simulink model "queuetest_third"  (R2018a)
settings: Solver=FixedStepDiscrete  StartTime=0.0  StopTime=10  RelTol=1e-3  EnableMultiTasking=on
model workspace (MAT data in the model file):
  deltat = 0.001
libraries: dspbuff3 x1
settings Model: Creator=The MathWorks, Inc.  LastModifiedBy=Michael Girbino
settings SolverCC: InsertRTBMode=Auto
settings DataIOCC: LimitDataPoints=on  SaveFormat=Array
settings OptimizationCC: ExpressionDepthLimit=2147483647  InitFltsAndDblsToZero=on  LifeSpan=inf
settings DebuggingCC: SaveWithParameterizedLinksMsg=none  UnderspecifiedInitializationDetection=Classic  MergeDetectMultiDrivingBlocksExec=none  SignalResolutionControl=TryResolveAllWithWarning  InheritedTsInSrcMsg=none  MultiTaskDSMMsg=warning  MultiTaskCondExecSysMsg=none  FcnCallInpInsideContextMsg=warning  StateNameClashWarn=warning  SFUnexpectedBacktrackingDiag=warning  SFNoUnconditionalDefaultTransitionDiag=warning  SFExecutionAtInitializationDiag=none
settings HardwareCC: ProdBitPerPointer=32  ProdBitPerSizeT=32  ProdBitPerPtrDiffT=32  ProdLargestAtomicFloat=None  ProdIntDivRoundTo=Undefined  ProdEndianess=Unspecified  ProdWordSize=32  ProdHWDeviceType=32-bit Generic
settings ModelReferenceCC: PropagateSignalLabelsOutOfModel=off
settings SFSimCC: SFSimEcho=off  SimParseCustomCode=off
settings CodeAppCC: StateflowObjectComments=on
settings GRTTargetCC: TargetFcnLib=ansi_tfl_tmw.mat  TargetLangStandard=C89/C90 (ANSI)  GeneratePreprocessorConditionals=Disable all  CombineOutputUpdateFcns=off  GRTInterface=on
settings ConfigComp: CovMetricSettings=dw  CovHtmlReporting=on  CovSaveCumulativeToWorkspaceVar=on  CovSaveSingleToWorkspaceVar=on  CovExternalEMLEnable=off  CovSFcnEnable=off

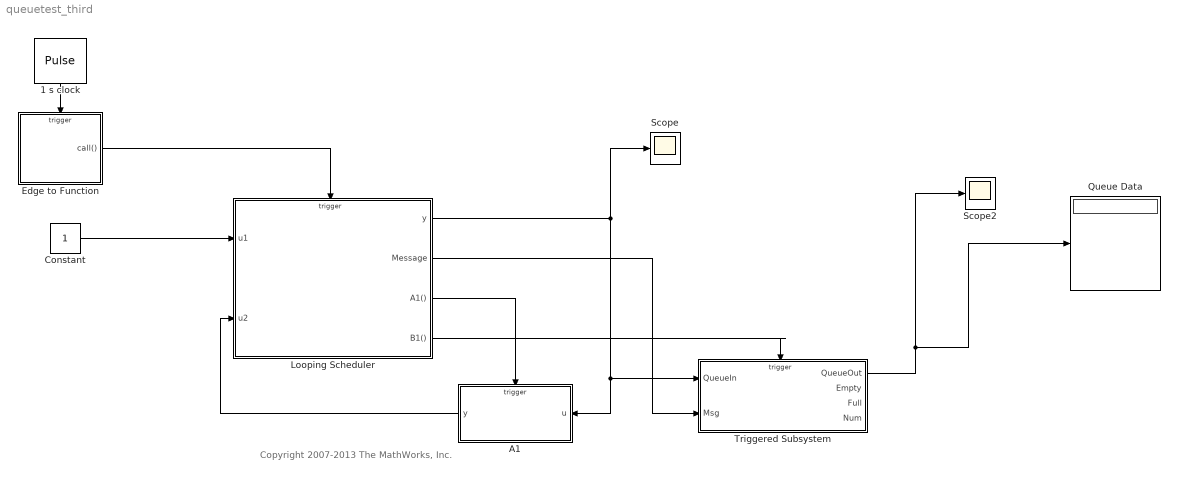
== system queuetest_third ==
  note: Copyright 2007-2013 The MathWorks, Inc.
  1 s clock : DiscretePulseGenerator  PulseType=Time based  Period=1  PulseWidth=10
  A1 : Subsystem  TreatAsAtomicUnit=on
  Constant : Constant
  "Edge to Function " : Stateflow chart  TreatAsAtomicUnit=on
  Looping Scheduler : Stateflow chart  TreatAsAtomicUnit=on
  Queue Data : Display
  Scope : Scope
  Scope2 : Scope
  Triggered Subsystem : Subsystem  TreatAsAtomicUnit=on
  wires:
  Looping Scheduler/1(y) -> Triggered Subsystem/1(QueueIn), A1/1(u), Scope/1
  Looping Scheduler/3(A1()) -> A1/Trigger
  A1/1(y) -> Looping Scheduler/2(u2)
  Constant/1 -> Looping Scheduler/1(u1)
  1 s clock/1 -> "Edge to Function "/Trigger
  "Edge to Function "/1(call()) -> Looping Scheduler/Trigger
  Triggered Subsystem/1(QueueOut) -> Queue Data/1, Scope2/1
  Looping Scheduler/4(B1()) -> Triggered Subsystem/Trigger
  Looping Scheduler/2(Message) -> Triggered Subsystem/2(Msg)

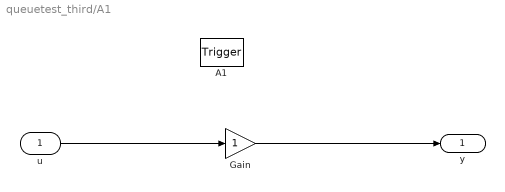
== system queuetest_third/A1 ==
  u : Inport
  A1 : TriggerPort  TriggerType=function-call  VariantControl=Variant
  Gain : Gain
  y : Outport
  wires:
  u/1 -> Gain/1
  Gain/1 -> y/1

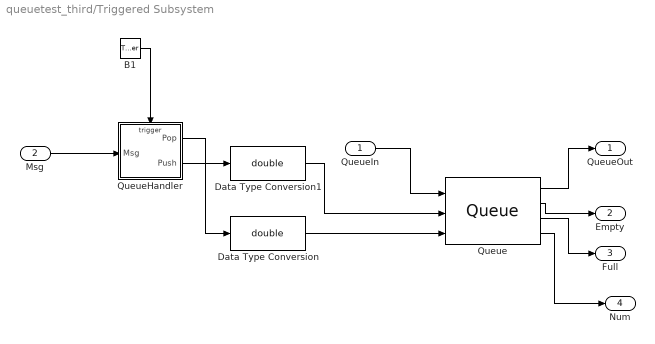
== system queuetest_third/Triggered Subsystem ==
  QueueIn : Inport  OutDataTypeStr=double
  Msg : Inport  Port=2  OutDataTypeStr=double
  B1 : TriggerPort  TriggerType=function-call  VariantControl=Variant  ShowOutputPort=on  OutputDataType=int8  PortDimensions=1
  Data Type Conversion : DataTypeConversion  OutDataTypeStr=double
  Data Type Conversion1 : DataTypeConversion  OutDataTypeStr=double
  Queue : dspbuff3/Queue  depth=8  trigger=Either edge  overflow=Dynamic reallocation  pes=Warning  eso=on  fso=on  nso=on  clr=off  clrOutport=off  adf=on
      settings: SourceProductName=DSP System Toolbox  SourceProductBaseCode=DS
  QueueHandler : Stateflow chart  TreatAsAtomicUnit=on
  QueueOut : Outport  OutDataTypeStr=double
  Empty : Outport  Port=2  OutDataTypeStr=boolean
  Full : Outport  Port=3  OutDataTypeStr=boolean
  Num : Outport  Port=4  OutDataTypeStr=double
  wires:
  QueueIn/1 -> Queue/1
  Queue/1 -> QueueOut/1
  Queue/2 -> Empty/1
  Queue/3 -> Full/1
  Queue/4 -> Num/1
  QueueHandler/1(Pop) -> Data Type Conversion/1
  Data Type Conversion/1 -> Queue/3
  Msg/1 -> QueueHandler/1(Msg)
  B1/1 -> QueueHandler/Trigger
  QueueHandler/2(Push) -> Data Type Conversion1/1
  Data Type Conversion1/1 -> Queue/2

== stateflow chart queuetest_third/Looping Scheduler ==
  (default) -> (junction 5) : {i=1;}
  (junction 6) -> (junction 5) [order 1] : [i<=10]
      | {
      |  y = u1+u2;
      | Message = 1;
      | send(A1);
      | send(B1);
      | i++;
      | }
  (junction 5) -> (junction 6)
  (junction 6) -> (junction 7) [order 2] : // done
  data: y output double; u1 input; u2 input; i local uint32; Message output double
  events: A1 output FUNCTION_CALL_EVENT; call input FUNCTION_CALL_EVENT; B1 output FUNCTION_CALL_EVENT

== stateflow chart queuetest_third/Edge to Function  ==
  (default) -> (junction 2) : {call;}
  events: edge input RISING_EDGE_EVENT; call output FUNCTION_CALL_EVENT

== stateflow chart queuetest_third/Triggered Subsystem/QueueHandler ==
  (default) -> (junction 19)
  (junction 19) -> (junction 20) [order 1] : [Msg == 1]
  (junction 19) -> (junction 21) [order 2]
  (junction 20) -> (junction 25) : {send(Push);}
  (junction 21) -> (junction 22) [order 1] : [Msg == 2]
  (junction 21) -> (junction 23) [order 2]
  (junction 22) -> (junction 24) : {send(Pop);}
  (junction 24) -> (junction 23)
  (junction 25) -> (junction 24)
  (junction 23) -> (junction 26)
  data: Msg input double
  events: Pop output EITHER_EDGE_EVENT; Push output EITHER_EDGE_EVENT; Run input EITHER_EDGE_EVENT
